simulink subsystem "REGISTERS_10_SS"  (R2022a)
settings: Solver=VariableStepAuto  StartTime=0.0  StopTime=10.0  RelTol=1e-3
libraries: hdlBasic x6395
(part 1 of 23)
settings Model: Creator=sebas  LastModifiedBy=viktor

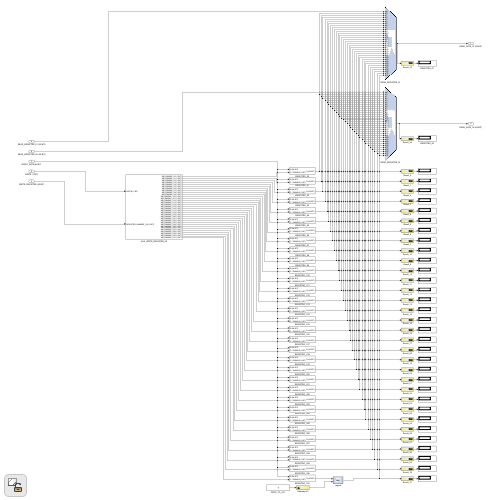
[thumbnail: Simulink's stored preview of the top-level diagram]
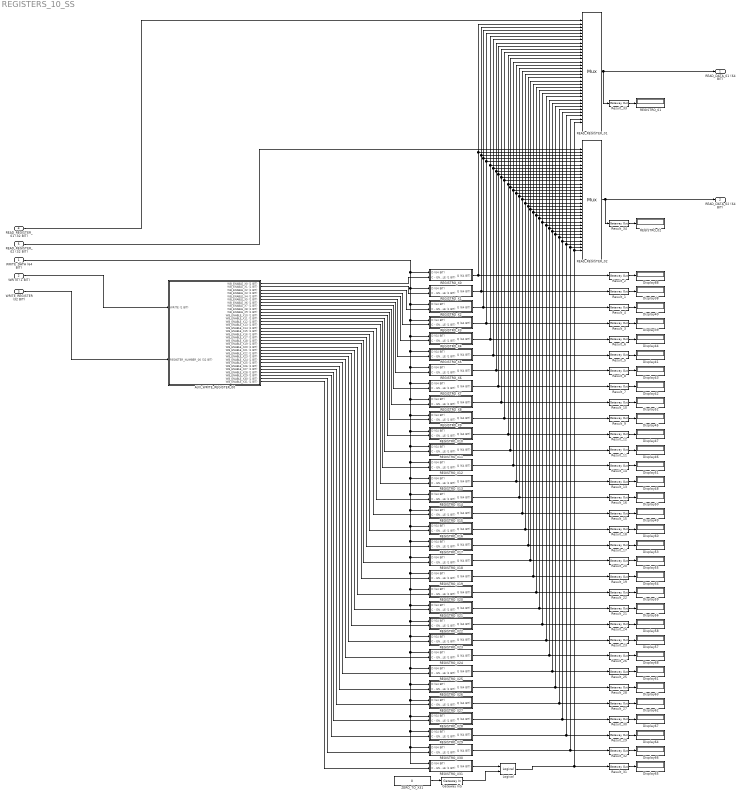
== system REGISTERS_10_SS ==
  WRITE_DATA (64 BIT) : Inport
  WRITE (1 BIT) : Inport  Port=2
  WRITE_REGISTER (32 BIT) : Inport  Port=3
  READ_REGISTER_01 (32 BIT) : Inport  Port=4
  READ_REGISTER_02 (32 BIT) : Inport  Port=5
  AUX_WRITE_REGISTER_00 : Subsystem
  Display{38..68,88} (32 alike) : Display
      settings: Format=decimal (Stored Integer)
  Gateway In5 : hdlBasic/Gateway In  gui_display_data_type=Fixed-point  arith_type=Signed (2's comp)  n_bits=64  bin_pt=0  preci_type=Single  exp_width=8  frac_width=24  rows=1  columns=1  quantization="Round  (unbiased: +/- Inf)"  overflow=Saturate  period=1  UseAsADC=off  ADCChannel='1'  interface=None  automatic_assignment=on  address_offset=hex2dec('00')  intf_name=''  intf_description=''  default_value=0  timing_constraint=None  locs_specified=off  LOCs={}  io_standard={}  inherit_from_input=off  hdl_port=on  XmcBlockStatus=1  maskContainerNames=group4  block_type=gatewayin  block_config=sysgen:gateway_in_config  block_width_w=590  block_height_w=620  block_width=640  block_height=850
  Logical : hdlBasic/Logical  logical_function=AND  inputs=2  en=off  latency=0  precision=Full  arith_type=Unsigned  n_bits=16  bin_pt=0  align_bp=on  overflow=[]  quantization=[]  XmcBlockStatus=1  maskContainerNames=tabcontainer1  block_type=logical  block_config=sysgen:Logical_config
  READ_REGISTER_01 : hdlBasic/Mux  inputs=32  en=off  latency=0  precision=Full  arith_type=Unsigned  n_bits=16  bin_pt=14  quantization=Truncate  overflow=Wrap  XmcBlockStatus=1  maskContainerNames=tabcontainer1  block_type=mux  block_config=sysgen:Mux_config
  READ_REGISTER_02 : hdlBasic/Mux  inputs=32  en=off  latency=0  precision=Full  arith_type=Unsigned  n_bits=16  bin_pt=14  quantization=Truncate  overflow=Wrap  XmcBlockStatus=1  maskContainerNames=tabcontainer1  block_type=mux  block_config=sysgen:Mux_config
  REGISTRO_01 : Display
      settings: Format=decimal (Stored Integer)
  REGISTRO_02 : Display
      settings: Format=decimal (Stored Integer)
  REGISTRO_X0 : Subsystem
  REGISTRO_X1 : Subsystem
  REGISTRO_X10 : Subsystem
  REGISTRO_X11 : Subsystem
  REGISTRO_X12 : Subsystem
  REGISTRO_X13 : Subsystem
  REGISTRO_X14 : Subsystem
  REGISTRO_X15 : Subsystem
  REGISTRO_X16 : Subsystem
  REGISTRO_X17 : Subsystem
  REGISTRO_X18 : Subsystem
  REGISTRO_X19 : Subsystem
  REGISTRO_X2 : Subsystem
  REGISTRO_X20 : Subsystem
  REGISTRO_X21 : Subsystem
  REGISTRO_X22 : Subsystem
  REGISTRO_X23 : Subsystem
  REGISTRO_X24 : Subsystem
  REGISTRO_X25 : Subsystem
  REGISTRO_X26 : Subsystem
  REGISTRO_X27 : Subsystem
  REGISTRO_X28 : Subsystem
  REGISTRO_X29 : Subsystem
  REGISTRO_X3 : Subsystem
  REGISTRO_X30 : Subsystem
  REGISTRO_X31 : Subsystem
  REGISTRO_X4 : Subsystem
  REGISTRO_X5 : Subsystem
  REGISTRO_X6 : Subsystem
  REGISTRO_X7 : Subsystem
  REGISTRO_X8 : Subsystem
  REGISTRO_X9 : Subsystem
  Result_{1..34} (34 alike) : hdlBasic/Gateway Out  inherit_from_input=off  hdl_port=on  rows=1  columns=1  UseAsDAC=off  DACChannel='1'  interface=None  automatic_assignment=on  address_offset=hex2dec('00')  intf_name=''  intf_description=''  timing_constraint=None  locs_specified=off  LOCs={}  io_standard={}  XmcBlockStatus=1  maskContainerNames=group4  block_type=gatewayout  block_config=sysgen:gateway_out_config  block_width_w=590  block_height_w=620  block_width=620  block_height=750
  ZERO_TO_X31 : Constant  Value=0
  READ_DATA_01 (64 BIT) : Outport
  READ_DATA_02 (64 BIT) : Outport  Port=2
  wires:
  REGISTRO_X11/1(Q (64 BIT)) -> Result_11/1, READ_REGISTER_02/13, READ_REGISTER_01/13
  AUX_WRITE_REGISTER_00/26(WB_ENABLE_X25 (1 BIT)) -> REGISTRO_X25/2(C - ENABLE (1 BIT))
  REGISTRO_X14/1(Q (64 BIT)) -> Result_16/1, READ_REGISTER_02/16, READ_REGISTER_01/16
  REGISTRO_X2/1(Q (64 BIT)) -> Result_4/1, READ_REGISTER_02/4, READ_REGISTER_01/4
  REGISTRO_X13/1(Q (64 BIT)) -> Result_13/1, READ_REGISTER_02/15, READ_REGISTER_01/15
  AUX_WRITE_REGISTER_00/10(WB_ENABLE_X9 (1 BIT)) -> REGISTRO_X9/2(C - ENABLE (1 BIT))
  REGISTRO_X1/1(Q (64 BIT)) -> Result_1/1, READ_REGISTER_02/3, READ_REGISTER_01/3
  AUX_WRITE_REGISTER_00/17(WB_ENABLE_X16 (1 BIT)) -> REGISTRO_X16/2(C - ENABLE (1 BIT))
  Result_7/1 -> Display42/1
  ZERO_TO_X31/1 -> Gateway In5/1
  Gateway In5/1 -> Logical/2
  REGISTRO_X8/1(Q (64 BIT)) -> Result_10/1, READ_REGISTER_02/10, READ_REGISTER_01/10
  AUX_WRITE_REGISTER_00/13(WB_ENABLE_X12 (1 BIT)) -> REGISTRO_X12/2(C - ENABLE (1 BIT))
  Result_28/1 -> Display63/1
  WRITE_DATA (64 BIT)/1 -> REGISTRO_X0/1(D (64 BIT)), REGISTRO_X1/1(D (64 BIT)), REGISTRO_X2/1(D (64 BIT)), REGISTRO_X3/1(D (64 BIT)), REGISTRO_X4/1(D (64 BIT)), REGISTRO_X30/1(D (64 BIT)), REGISTRO_X31/1(D (64 BIT)), REGISTRO_X29/1(D (64 BIT)), REGISTRO_X28/1(D (64 BIT)), REGISTRO_X27/1(D (64 BIT)), REGISTRO_X26/1(D (64 BIT)), REGISTRO_X25/1(D (64 BIT)), REGISTRO_X24/1(D (64 BIT)), REGISTRO_X23/1(D (64 BIT)), REGISTRO_X22/1(D (64 BIT)), REGISTRO_X21/1(D (64 BIT)), REGISTRO_X20/1(D (64 BIT)), REGISTRO_X19/1(D (64 BIT)), REGISTRO_X18/1(D (64 BIT)), REGISTRO_X17/1(D (64 BIT)), REGISTRO_X16/1(D (64 BIT)), REGISTRO_X15/1(D (64 BIT)), REGISTRO_X14/1(D (64 BIT)), REGISTRO_X13/1(D (64 BIT)), REGISTRO_X12/1(D (64 BIT)), REGISTRO_X11/1(D (64 BIT)), REGISTRO_X10/1(D (64 BIT)), REGISTRO_X9/1(D (64 BIT)), REGISTRO_X8/1(D (64 BIT)), REGISTRO_X7/1(D (64 BIT)), REGISTRO_X6/1(D (64 BIT)), REGISTRO_X5/1(D (64 BIT))
  Result_24/1 -> Display58/1
  AUX_WRITE_REGISTER_00/32(WB_ENABLE_X31 (1 BIT)) -> REGISTRO_X31/2(C - ENABLE (1 BIT))
  REGISTRO_X23/1(Q (64 BIT)) -> Result_23/1, READ_REGISTER_02/25, READ_REGISTER_01/25
  REGISTRO_X0/1(Q (64 BIT)) -> Result_2/1, READ_REGISTER_02/2, READ_REGISTER_01/2
  AUX_WRITE_REGISTER_00/21(WB_ENABLE_X20 (1 BIT)) -> REGISTRO_X20/2(C - ENABLE (1 BIT))
  Result_25/1 -> Display61/1
  REGISTRO_X12/1(Q (64 BIT)) -> Result_14/1, READ_REGISTER_02/14, READ_REGISTER_01/14
  AUX_WRITE_REGISTER_00/20(WB_ENABLE_X19 (1 BIT)) -> REGISTRO_X19/2(C - ENABLE (1 BIT))
  REGISTRO_X21/1(Q (64 BIT)) -> Result_21/1, READ_REGISTER_02/23, READ_REGISTER_01/23
  REGISTRO_X28/1(Q (64 BIT)) -> Result_30/1, READ_REGISTER_02/30, READ_REGISTER_01/30
  Result_5/1 -> Display41/1
  Logical/1 -> Result_31/1, READ_REGISTER_02/33, READ_REGISTER_01/33
  REGISTRO_X5/1(Q (64 BIT)) -> Result_5/1, READ_REGISTER_02/7, READ_REGISTER_01/7
  WRITE (1 BIT)/1 -> AUX_WRITE_REGISTER_00/1(WRITE (1 BIT))
  AUX_WRITE_REGISTER_00/24(WB_ENABLE_X23 (1 BIT)) -> REGISTRO_X23/2(C - ENABLE (1 BIT))
  AUX_WRITE_REGISTER_00/19(WB_ENABLE_X18 (1 BIT)) -> REGISTRO_X18/2(C - ENABLE (1 BIT))
  Result_12/1 -> Display47/1
  REGISTRO_X15/1(Q (64 BIT)) -> Result_15/1, READ_REGISTER_02/17, READ_REGISTER_01/17
  REGISTRO_X29/1(Q (64 BIT)) -> Result_29/1, READ_REGISTER_02/31, READ_REGISTER_01/31
  AUX_WRITE_REGISTER_00/29(WB_ENABLE_X28 (1 BIT)) -> REGISTRO_X28/2(C - ENABLE (1 BIT))
  REGISTRO_X31/1(Q (64 BIT)) -> Logical/1
  AUX_WRITE_REGISTER_00/16(WB_ENABLE_X15 (1 BIT)) -> REGISTRO_X15/2(C - ENABLE (1 BIT))
  AUX_WRITE_REGISTER_00/18(WB_ENABLE_X17 (1 BIT)) -> REGISTRO_X17/2(C - ENABLE (1 BIT))
  AUX_WRITE_REGISTER_00/28(WB_ENABLE_X27 (1 BIT)) -> REGISTRO_X27/2(C - ENABLE (1 BIT))
  REGISTRO_X3/1(Q (64 BIT)) -> Result_3/1, READ_REGISTER_02/5, READ_REGISTER_01/5
  AUX_WRITE_REGISTER_00/31(WB_ENABLE_X30 (1 BIT)) -> REGISTRO_X30/2(C - ENABLE (1 BIT))
  AUX_WRITE_REGISTER_00/12(WB_ENABLE_X11 (1 BIT)) -> REGISTRO_X11/2(C - ENABLE (1 BIT))
  REGISTRO_X19/1(Q (64 BIT)) -> Result_19/1, READ_REGISTER_02/21, READ_REGISTER_01/21
  AUX_WRITE_REGISTER_00/27(WB_ENABLE_X26 (1 BIT)) -> REGISTRO_X26/2(C - ENABLE (1 BIT))
  Result_31/1 -> Display65/1
  REGISTRO_X30/1(Q (64 BIT)) -> Result_32/1, READ_REGISTER_02/32, READ_REGISTER_01/32
  Result_23/1 -> Display57/1
  AUX_WRITE_REGISTER_00/11(WB_ENABLE_X10 (1 BIT)) -> REGISTRO_X10/2(C - ENABLE (1 BIT))
  Result_18/1 -> Display60/1
  Result_6/1 -> Display44/1
  Result_22/1 -> Display59/1
  REGISTRO_X20/1(Q (64 BIT)) -> Result_22/1, READ_REGISTER_02/22, READ_REGISTER_01/22
  Result_26/1 -> Display68/1
  REGISTRO_X18/1(Q (64 BIT)) -> Result_20/1, READ_REGISTER_02/20, READ_REGISTER_01/20
  Result_33/1 -> REGISTRO_01/1
  REGISTRO_X6/1(Q (64 BIT)) -> Result_8/1, READ_REGISTER_02/8, READ_REGISTER_01/8
  Result_19/1 -> Display54/1
  REGISTRO_X17/1(Q (64 BIT)) -> Result_17/1, READ_REGISTER_02/19, READ_REGISTER_01/19
  Result_21/1 -> Display56/1
  AUX_WRITE_REGISTER_00/15(WB_ENABLE_X14 (1 BIT)) -> REGISTRO_X14/2(C - ENABLE (1 BIT))
  Result_29/1 -> Display64/1
  REGISTRO_X26/1(Q (64 BIT)) -> Result_28/1, READ_REGISTER_02/28, READ_REGISTER_01/28
  REGISTRO_X27/1(Q (64 BIT)) -> Result_27/1, READ_REGISTER_02/29, READ_REGISTER_01/29
  REGISTRO_X25/1(Q (64 BIT)) -> Result_25/1, READ_REGISTER_02/27, READ_REGISTER_01/27
  Result_15/1 -> Display49/1
  REGISTRO_X24/1(Q (64 BIT)) -> Result_26/1, READ_REGISTER_02/26, READ_REGISTER_01/26
  READ_REGISTER_02/1 -> Result_34/1, READ_DATA_02 (64 BIT)/1
  Result_14/1 -> Display51/1
  Result_27/1 -> Display62/1
  REGISTRO_X7/1(Q (64 BIT)) -> Result_7/1, READ_REGISTER_02/9, READ_REGISTER_01/9
  Result_4/1 -> Display40/1
  REGISTRO_X4/1(Q (64 BIT)) -> Result_6/1, READ_REGISTER_02/6, READ_REGISTER_01/6
  Result_17/1 -> Display53/1
  Result_16/1 -> Display50/1
  Result_20/1 -> Display55/1
  Result_32/1 -> Display66/1
  REGISTRO_X9/1(Q (64 BIT)) -> Result_9/1, READ_REGISTER_02/11, READ_REGISTER_01/11
  Result_30/1 -> Display67/1
  READ_REGISTER_02 (32 BIT)/1 -> READ_REGISTER_02/1
  Result_3/1 -> Display39/1
  AUX_WRITE_REGISTER_00/3(WB_ENABLE_X2 (1 BIT)) -> REGISTRO_X2/2(C - ENABLE (1 BIT))
  Result_10/1 -> Display52/1
  REGISTRO_X10/1(Q (64 BIT)) -> Result_12/1, READ_REGISTER_02/12, READ_REGISTER_01/12
  AUX_WRITE_REGISTER_00/4(WB_ENABLE_X3 (1 BIT)) -> REGISTRO_X3/2(C - ENABLE (1 BIT))
  Result_1/1 -> Display38/1
  REGISTRO_X16/1(Q (64 BIT)) -> Result_18/1, READ_REGISTER_02/18, READ_REGISTER_01/18
  Result_2/1 -> Display88/1
  AUX_WRITE_REGISTER_00/2(WB_ENABLE_X1 (1 BIT)) -> REGISTRO_X1/2(C - ENABLE (1 BIT))
  AUX_WRITE_REGISTER_00/14(WB_ENABLE_X13 (1 BIT)) -> REGISTRO_X13/2(C - ENABLE (1 BIT))
  AUX_WRITE_REGISTER_00/6(WB_ENABLE_X5 (1 BIT)) -> REGISTRO_X5/2(C - ENABLE (1 BIT))
  Result_13/1 -> Display48/1
  AUX_WRITE_REGISTER_00/1(WB_ENABLE_X0 (1 BIT)) -> REGISTRO_X0/2(C - ENABLE (1 BIT))
  Result_9/1 -> Display45/1
  READ_REGISTER_01/1 -> Result_33/1, READ_DATA_01 (64 BIT)/1
  REGISTRO_X22/1(Q (64 BIT)) -> Result_24/1, READ_REGISTER_02/24, READ_REGISTER_01/24
  WRITE_REGISTER (32 BIT)/1 -> AUX_WRITE_REGISTER_00/2(REGISTER_NUMBER_00 (32 BIT))
  AUX_WRITE_REGISTER_00/9(WB_ENABLE_X8 (1 BIT)) -> REGISTRO_X8/2(C - ENABLE (1 BIT))
  AUX_WRITE_REGISTER_00/22(WB_ENABLE_X21 (1 BIT)) -> REGISTRO_X21/2(C - ENABLE (1 BIT))
  Result_34/1 -> REGISTRO_02/1
  AUX_WRITE_REGISTER_00/25(WB_ENABLE_X24 (1 BIT)) -> REGISTRO_X24/2(C - ENABLE (1 BIT))
  Result_8/1 -> Display43/1
  Result_11/1 -> Display46/1
  AUX_WRITE_REGISTER_00/7(WB_ENABLE_X6 (1 BIT)) -> REGISTRO_X6/2(C - ENABLE (1 BIT))
  AUX_WRITE_REGISTER_00/5(WB_ENABLE_X4 (1 BIT)) -> REGISTRO_X4/2(C - ENABLE (1 BIT))
  AUX_WRITE_REGISTER_00/8(WB_ENABLE_X7 (1 BIT)) -> REGISTRO_X7/2(C - ENABLE (1 BIT))
  AUX_WRITE_REGISTER_00/23(WB_ENABLE_X22 (1 BIT)) -> REGISTRO_X22/2(C - ENABLE (1 BIT))
  AUX_WRITE_REGISTER_00/30(WB_ENABLE_X29 (1 BIT)) -> REGISTRO_X29/2(C - ENABLE (1 BIT))
  READ_REGISTER_01 (32 BIT)/1 -> READ_REGISTER_01/1

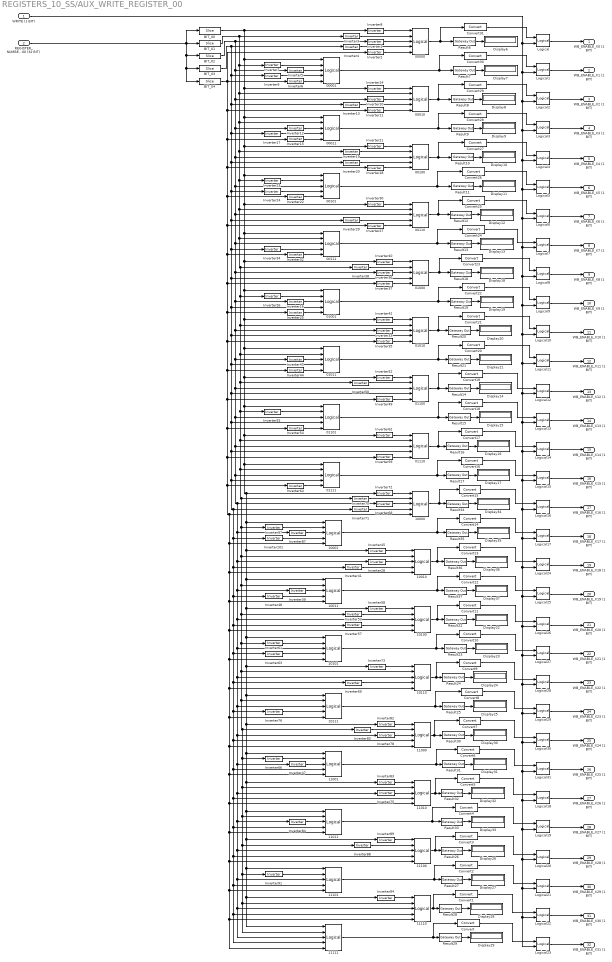
== system REGISTERS_10_SS/AUX_WRITE_REGISTER_00 ==
  WRITE (1 BIT) : Inport
  REGISTER_NUMBER_00 (32 BIT) : Inport  Port=2
  00000 : hdlBasic/Logical  logical_function=AND  inputs=5  en=off  latency=0  precision=Full  arith_type=Unsigned  n_bits=16  bin_pt=0  align_bp=on  overflow=[]  quantization=[]  XmcBlockStatus=1  maskContainerNames=tabcontainer1  block_type=logical  block_config=sysgen:Logical_config
  00001 : hdlBasic/Logical  logical_function=AND  inputs=5  en=off  latency=0  precision=Full  arith_type=Unsigned  n_bits=16  bin_pt=0  align_bp=on  overflow=[]  quantization=[]  XmcBlockStatus=1  maskContainerNames=tabcontainer1  block_type=logical  block_config=sysgen:Logical_config
  00010 : hdlBasic/Logical  logical_function=AND  inputs=5  en=off  latency=0  precision=Full  arith_type=Unsigned  n_bits=16  bin_pt=0  align_bp=on  overflow=[]  quantization=[]  XmcBlockStatus=1  maskContainerNames=tabcontainer1  block_type=logical  block_config=sysgen:Logical_config
  00011 : hdlBasic/Logical  logical_function=AND  inputs=5  en=off  latency=0  precision=Full  arith_type=Unsigned  n_bits=16  bin_pt=0  align_bp=on  overflow=[]  quantization=[]  XmcBlockStatus=1  maskContainerNames=tabcontainer1  block_type=logical  block_config=sysgen:Logical_config
  00100 : hdlBasic/Logical  logical_function=AND  inputs=5  en=off  latency=0  precision=Full  arith_type=Unsigned  n_bits=16  bin_pt=0  align_bp=on  overflow=[]  quantization=[]  XmcBlockStatus=1  maskContainerNames=tabcontainer1  block_type=logical  block_config=sysgen:Logical_config
  00101 : hdlBasic/Logical  logical_function=AND  inputs=5  en=off  latency=0  precision=Full  arith_type=Unsigned  n_bits=16  bin_pt=0  align_bp=on  overflow=[]  quantization=[]  XmcBlockStatus=1  maskContainerNames=tabcontainer1  block_type=logical  block_config=sysgen:Logical_config
  00110 : hdlBasic/Logical  logical_function=AND  inputs=5  en=off  latency=0  precision=Full  arith_type=Unsigned  n_bits=16  bin_pt=0  align_bp=on  overflow=[]  quantization=[]  XmcBlockStatus=1  maskContainerNames=tabcontainer1  block_type=logical  block_config=sysgen:Logical_config
  00111 : hdlBasic/Logical  logical_function=AND  inputs=5  en=off  latency=0  precision=Full  arith_type=Unsigned  n_bits=16  bin_pt=0  align_bp=on  overflow=[]  quantization=[]  XmcBlockStatus=1  maskContainerNames=tabcontainer1  block_type=logical  block_config=sysgen:Logical_config
  01000 : hdlBasic/Logical  logical_function=AND  inputs=5  en=off  latency=0  precision=Full  arith_type=Unsigned  n_bits=16  bin_pt=0  align_bp=on  overflow=[]  quantization=[]  XmcBlockStatus=1  maskContainerNames=tabcontainer1  block_type=logical  block_config=sysgen:Logical_config
  01001 : hdlBasic/Logical  logical_function=AND  inputs=5  en=off  latency=0  precision=Full  arith_type=Unsigned  n_bits=16  bin_pt=0  align_bp=on  overflow=[]  quantization=[]  XmcBlockStatus=1  maskContainerNames=tabcontainer1  block_type=logical  block_config=sysgen:Logical_config
  01010 : hdlBasic/Logical  logical_function=AND  inputs=5  en=off  latency=0  precision=Full  arith_type=Unsigned  n_bits=16  bin_pt=0  align_bp=on  overflow=[]  quantization=[]  XmcBlockStatus=1  maskContainerNames=tabcontainer1  block_type=logical  block_config=sysgen:Logical_config
  01011 : hdlBasic/Logical  logical_function=AND  inputs=5  en=off  latency=0  precision=Full  arith_type=Unsigned  n_bits=16  bin_pt=0  align_bp=on  overflow=[]  quantization=[]  XmcBlockStatus=1  maskContainerNames=tabcontainer1  block_type=logical  block_config=sysgen:Logical_config
  01100 : hdlBasic/Logical  logical_function=AND  inputs=5  en=off  latency=0  precision=Full  arith_type=Unsigned  n_bits=16  bin_pt=0  align_bp=on  overflow=[]  quantization=[]  XmcBlockStatus=1  maskContainerNames=tabcontainer1  block_type=logical  block_config=sysgen:Logical_config
  01101 : hdlBasic/Logical  logical_function=AND  inputs=5  en=off  latency=0  precision=Full  arith_type=Unsigned  n_bits=16  bin_pt=0  align_bp=on  overflow=[]  quantization=[]  XmcBlockStatus=1  maskContainerNames=tabcontainer1  block_type=logical  block_config=sysgen:Logical_config
  01110 : hdlBasic/Logical  logical_function=AND  inputs=5  en=off  latency=0  precision=Full  arith_type=Unsigned  n_bits=16  bin_pt=0  align_bp=on  overflow=[]  quantization=[]  XmcBlockStatus=1  maskContainerNames=tabcontainer1  block_type=logical  block_config=sysgen:Logical_config
  01111 : hdlBasic/Logical  logical_function=AND  inputs=5  en=off  latency=0  precision=Full  arith_type=Unsigned  n_bits=16  bin_pt=0  align_bp=on  overflow=[]  quantization=[]  XmcBlockStatus=1  maskContainerNames=tabcontainer1  block_type=logical  block_config=sysgen:Logical_config
  {10000..10001,10010..10011,10100..10101,10110..10111,11000..11001,11010..11011,11100..11101,11110..11111} (16 alike) : hdlBasic/Logical  logical_function=AND  inputs=5  en=off  latency=0  precision=Full  arith_type=Unsigned  n_bits=16  bin_pt=0  align_bp=on  overflow=[]  quantization=[]  XmcBlockStatus=1  maskContainerNames=tabcontainer1  block_type=logical  block_config=sysgen:Logical_config
  BIT_00 : hdlBasic/Slice  nbits=1  boolean_output=off  mode=Lower Bit Location + Width  bit1=-3  base1=MSB of Input  bit0=0  base0=LSB of Input  XmcBlockStatus=1  maskContainerNames=group1  block_type=slice  block_config=sysgen:Slice_config
  BIT_01 : hdlBasic/Slice  nbits=1  boolean_output=off  mode=Lower Bit Location + Width  bit1=-2  base1=MSB of Input  bit0=1  base0=LSB of Input  XmcBlockStatus=1  maskContainerNames=group1  block_type=slice  block_config=sysgen:Slice_config
  BIT_02 : hdlBasic/Slice  nbits=1  boolean_output=off  mode=Lower Bit Location + Width  bit1=-3  base1=MSB of Input  bit0=2  base0=LSB of Input  XmcBlockStatus=1  maskContainerNames=group1  block_type=slice  block_config=sysgen:Slice_config
  BIT_03 : hdlBasic/Slice  nbits=1  boolean_output=off  mode=Lower Bit Location + Width  bit1=-2  base1=MSB of Input  bit0=3  base0=LSB of Input  XmcBlockStatus=1  maskContainerNames=group1  block_type=slice  block_config=sysgen:Slice_config
  BIT_04 : hdlBasic/Slice  nbits=1  boolean_output=off  mode=Lower Bit Location + Width  bit1=-2  base1=MSB of Input  bit0=4  base0=LSB of Input  XmcBlockStatus=1  maskContainerNames=group1  block_type=slice  block_config=sysgen:Slice_config
  Convert{,1..31} (32 alike) : hdlBasic/Convert  gui_display_data_type=Boolean  arith_type=Boolean  n_bits=16  bin_pt=14  float_type=Single  exp_bits=8  fraction_bits=24  quantization=Truncate  overflow=Wrap  en=off  latency=0  pipeline=off  XmcBlockStatus=1  maskContainerNames=group2  block_type=convert  block_config=sysgen:Convert_config  block_width=595  block_height=885
  Display{6..37} (32 alike) : Display
  Inverter{1..30,32..45,47..50,52..55,57..59,61..64,66,68..73,75..76,78,80,82..84,87..89,91,94,97,101} (80 alike) : hdlBasic/Inverter  en=off  latency=0  XmcBlockStatus=1  maskContainerNames=group2  block_type=inv  block_config=sysgen:Inverter_config
  Logical{,1..31} (32 alike) : hdlBasic/Logical  logical_function=AND  inputs=2  en=off  latency=0  precision=Full  arith_type=Unsigned  n_bits=16  bin_pt=0  align_bp=on  overflow=[]  quantization=[]  XmcBlockStatus=1  maskContainerNames=tabcontainer1  block_type=logical  block_config=sysgen:Logical_config
  Result{6..37} (32 alike) : hdlBasic/Gateway Out  inherit_from_input=off  hdl_port=on  rows=1  columns=1  UseAsDAC=off  DACChannel='1'  interface=None  automatic_assignment=on  address_offset=hex2dec('00')  intf_name=''  intf_description=''  timing_constraint=None  locs_specified=off  LOCs={}  io_standard={}  XmcBlockStatus=1  maskContainerNames=group4  block_type=gatewayout  block_config=sysgen:gateway_out_config  block_width_w=590  block_height_w=620  block_width=620  block_height=750
  WB_ENABLE_X0 (1 BIT) : Outport
  WB_ENABLE_X1 (1 BIT) : Outport  Port=2
  WB_ENABLE_X2 (1 BIT) : Outport  Port=3
  WB_ENABLE_X3 (1 BIT) : Outport  Port=4
  WB_ENABLE_X4 (1 BIT) : Outport  Port=5
  WB_ENABLE_X5 (1 BIT) : Outport  Port=6
  WB_ENABLE_X6 (1 BIT) : Outport  Port=7
  WB_ENABLE_X7 (1 BIT) : Outport  Port=8
  WB_ENABLE_X8 (1 BIT) : Outport  Port=9
  WB_ENABLE_X9 (1 BIT) : Outport  Port=10
  WB_ENABLE_X10 (1 BIT) : Outport  Port=11
  WB_ENABLE_X11 (1 BIT) : Outport  Port=12
  WB_ENABLE_X12 (1 BIT) : Outport  Port=13
  WB_ENABLE_X13 (1 BIT) : Outport  Port=14
  WB_ENABLE_X14 (1 BIT) : Outport  Port=15
  WB_ENABLE_X15 (1 BIT) : Outport  Port=16
  WB_ENABLE_X16 (1 BIT) : Outport  Port=17
  WB_ENABLE_X17 (1 BIT) : Outport  Port=18
  WB_ENABLE_X18 (1 BIT) : Outport  Port=19
  WB_ENABLE_X19 (1 BIT) : Outport  Port=20
  WB_ENABLE_X20 (1 BIT) : Outport  Port=21
  WB_ENABLE_X21 (1 BIT) : Outport  Port=22
  WB_ENABLE_X22 (1 BIT) : Outport  Port=23
  WB_ENABLE_X23 (1 BIT) : Outport  Port=24
  WB_ENABLE_X24 (1 BIT) : Outport  Port=25
  WB_ENABLE_X25 (1 BIT) : Outport  Port=26
  WB_ENABLE_X26 (1 BIT) : Outport  Port=27
  WB_ENABLE_X27 (1 BIT) : Outport  Port=28
  WB_ENABLE_X28 (1 BIT) : Outport  Port=29
  WB_ENABLE_X29 (1 BIT) : Outport  Port=30
  WB_ENABLE_X30 (1 BIT) : Outport  Port=31
  WB_ENABLE_X31 (1 BIT) : Outport  Port=32
  wires:
  Logical3/1 -> WB_ENABLE_X3 (1 BIT)/1
  Inverter44/1 -> 01011/5
  Inverter88/1 -> 11100/2
  Result19/1 -> Display19/1
  Inverter6/1 -> 00001/5
  Convert18/1 -> Logical13/1
  00000/1 -> Result6/1, Convert31/1
  Result28/1 -> Display28/1
  Result7/1 -> Display7/1
  Inverter97/1 -> 10001/2
  Inverter41/1 -> 10010/4
  Convert19/1 -> Logical12/1
  Inverter43/1 -> 01011/3
  Inverter10/1 -> 00010/3
  Logical9/1 -> WB_ENABLE_X9 (1 BIT)/1
  Logical13/1 -> WB_ENABLE_X13 (1 BIT)/1
  Logical14/1 -> WB_ENABLE_X14 (1 BIT)/1
  Logical11/1 -> WB_ENABLE_X11 (1 BIT)/1
  Result22/1 -> Display22/1
  Inverter63/1 -> 10101/4
  Convert8/1 -> Logical29/1
  Inverter16/1 -> 01001/3
  Inverter66/1 -> 11001/2
  Convert5/1 -> Logical18/1
  Result12/1 -> Display12/1
  Inverter80/1 -> 11000/2
  Inverter17/1 -> 00011/4
  Result18/1 -> Display18/1
  Inverter8/1 -> 00000/1
  Result27/1 -> Display27/1
  Inverter34/1 -> 00111/4
  Result36/1 -> Display36/1
  11000/1 -> Result30/1, Convert7/1
  Logical/1 -> WB_ENABLE_X0 (1 BIT)/1
  Logical30/1 -> WB_ENABLE_X24 (1 BIT)/1
  Logical18/1 -> WB_ENABLE_X26 (1 BIT)/1
  Logical20/1 -> WB_ENABLE_X28 (1 BIT)/1
  Logical31/1 -> WB_ENABLE_X25 (1 BIT)/1
  Logical22/1 -> WB_ENABLE_X30 (1 BIT)/1
  Logical29/1 -> WB_ENABLE_X23 (1 BIT)/1
  Inverter38/1 -> 01000/2
  Logical24/1 -> WB_ENABLE_X18 (1 BIT)/1
  Logical1/1 -> WB_ENABLE_X1 (1 BIT)/1
  Inverter47/1 -> 11001/3
  01100/1 -> Result14/1, Convert19/1
  Result35/1 -> Display35/1
  Convert6/1 -> Logical31/1
  Convert4/1 -> Logical19/1
  Inverter83/1 -> 11010/1
  Convert3/1 -> Logical20/1
  10000/1 -> Result34/1, Convert15/1
  Inverter13/1 -> 00010/4
  Inverter75/1 -> 11010/3
  Convert11/1 -> Logical26/1
  Result29/1 -> Display29/1
  Inverter101/1 -> 10001/4
  Inverter72/1 -> 10000/1
  Inverter1/1 -> 00000/3
  Inverter3/1 -> 00000/2
  Convert15/1 -> Logical16/1
  Inverter14/1 -> 00010/1
  Inverter21/1 -> 00100/1
  Convert26/1 -> Logical5/1
  Inverter11/1 -> 00010/5
  Inverter58/1 -> 10100/1
  Result33/1 -> Display33/1
  Inverter36/1 -> 01000/3
  Inverter45/1 -> 10010/1
  Inverter9/1 -> 00001/4
  Inverter68/1 -> 10000/3
  01001/1 -> Result19/1, Convert22/1
  Logical21/1 -> WB_ENABLE_X29 (1 BIT)/1
  Convert9/1 -> Logical28/1
  Inverter25/1 -> 01001/5
  Result10/1 -> Display10/1
  Logical12/1 -> WB_ENABLE_X12 (1 BIT)/1
  Result11/1 -> Display11/1
  Result8/1 -> Display8/1
  Inverter5/1 -> 00001/3
  Inverter15/1 -> 00011/5
  Result25/1 -> Display25/1
  Result37/1 -> Display37/1
  Result16/1 -> Display16/1
  Result14/1 -> Display14/1
  Inverter59/1 -> 01110/5
  Convert14/1 -> Logical17/1
  Convert12/1 -> Logical25/1
  Logical17/1 -> WB_ENABLE_X17 (1 BIT)/1
  Convert10/1 -> Logical27/1
  Convert17/1 -> Logical14/1
  Inverter23/1 -> 00101/2
  Convert23/1 -> Logical8/1
  Convert30/1 -> Logical1/1
  Inverter24/1 -> 00101/4
  10111/1 -> Result25/1, Convert8/1
  Inverter20/1 -> 00100/4
  Inverter53/1 -> 10100/2
  Inverter73/1 -> 10110/1
  Convert22/1 -> Logical9/1
  Inverter7/1 -> 00001/2
  Inverter19/1 -> 00100/2
  01011/1 -> Result21/1, Convert20/1
  Convert13/1 -> Logical24/1
  Inverter84/1 -> 11011/3
  Result20/1 -> Display20/1
  Inverter48/1 -> 10011/4
  Inverter55/1 -> 01101/2
  Logical15/1 -> WB_ENABLE_X15 (1 BIT)/1
  10110/1 -> Result24/1, Convert9/1
  Result23/1 -> Display23/1
  Convert20/1 -> Logical11/1
  01000/1 -> Result18/1, Convert23/1
  11111/1 -> Result29/1, Convert/1
  Result17/1 -> Display17/1
  11110/1 -> Result28/1, Convert1/1
  01110/1 -> Result16/1, Convert17/1
  Inverter2/1 -> 00000/5
  Convert21/1 -> Logical10/1
  Inverter12/1 -> 00011/3
  Inverter27/1 -> 00110/5
  Convert1/1 -> Logical22/1
  Inverter37/1 -> 01000/5
  11101/1 -> Result27/1, Convert2/1
  Inverter32/1 -> 00111/5
  Inverter76/1 -> 10111/4
  Inverter62/1 -> 01110/1
  Inverter22/1 -> 00101/5
  01101/1 -> Result15/1, Convert18/1
  00100/1 -> Result10/1, Convert27/1
  10010/1 -> Result36/1, Convert13/1
  Result34/1 -> Display34/1
  Result9/1 -> Display9/1
  Inverter40/1 -> 01000/1
  Logical2/1 -> WB_ENABLE_X2 (1 BIT)/1
  Inverter87/1 -> 10001/3
  Inverter18/1 -> 00100/5
  Result15/1 -> Display15/1
  Inverter4/1 -> 00000/4
  01010/1 -> Result20/1, Convert21/1
  Inverter64/1 -> 01111/5
  Logical23/1 -> WB_ENABLE_X31 (1 BIT)/1
  Result24/1 -> Display24/1
  Inverter49/1 -> 01100/5
  00001/1 -> Result7/1, Convert30/1
  10101/1 -> Result23/1, Convert10/1
  Result32/1 -> Display32/1
  Inverter50/1 -> 01100/2
  REGISTER_NUMBER_00 (32 BIT)/1 -> BIT_01/1, BIT_04/1, BIT_03/1, BIT_02/1, BIT_00/1
  Inverter42/1 -> 01010/1
  Convert/1 -> Logical23/1
  Inverter71/1 -> 10000/4
  Inverter91/1 -> 11101/2
  Inverter70/1 -> 10000/2
  Convert31/1 -> Logical/1
  10100/1 -> Result22/1, Convert11/1
  Inverter28/1 -> 10010/3
  Inverter78/1 -> 11000/3
  Logical4/1 -> WB_ENABLE_X4 (1 BIT)/1
  Inverter89/1 -> 11100/1
  Inverter39/1 -> 10011/3
  Inverter82/1 -> 11000/1
  11011/1 -> Result33/1, Convert4/1
  Logical7/1 -> WB_ENABLE_X7 (1 BIT)/1
  Logical28/1 -> WB_ENABLE_X22 (1 BIT)/1
  Convert24/1 -> Logical7/1
  Inverter94/1 -> 11110/1
  10011/1 -> Result37/1, Convert12/1
  Convert16/1 -> Logical15/1
  Logical10/1 -> WB_ENABLE_X10 (1 BIT)/1
  Result21/1 -> Display21/1
  Logical19/1 -> WB_ENABLE_X27 (1 BIT)/1
  Inverter69/1 -> 10110/4
  Inverter61/1 -> 10101/2
  00010/1 -> Result8/1, Convert29/1
  00111/1 -> Result13/1, Convert24/1
  Result30/1 -> Display30/1
  Inverter29/1 -> 00110/4
  11100/1 -> Result26/1, Convert3/1
  Logical27/1 -> WB_ENABLE_X21 (1 BIT)/1
  BIT_02/1 -> Inverter1/1, Inverter5/1, 00100/3, 00101/3, 00110/3, 00111/3, Inverter36/1, Inverter16/1, Inverter33/1, Inverter43/1, 01100/3, 01101/3, Inverter68/1, Inverter87/1, 10100/3, 10101/3, 10110/3, 10111/3, Inverter78/1, Inverter47/1, Inverter75/1, Inverter84/1, 11100/3, 11101/3, 11111/3, 11110/3, Inverter39/1, Inverter28/1, 01111/3, 01110/3, Inverter12/1, Inverter10/1
  11001/1 -> Result31/1, Convert6/1
  Convert25/1 -> Logical6/1
  Logical5/1 -> WB_ENABLE_X5 (1 BIT)/1
  Inverter30/1 -> 00110/1
  Result6/1 -> Display6/1
  01111/1 -> Result17/1, Convert16/1
  10001/1 -> Result35/1, Convert14/1
  Inverter35/1 -> 01010/5
  00110/1 -> Result12/1, Convert25/1
  Inverter57/1 -> 10100/4
  Inverter54/1 -> 01101/5
  11010/1 -> Result32/1, Convert5/1
  Convert29/1 -> Logical2/1
  Inverter33/1 -> 01010/3
  BIT_04/1 -> Inverter6/1, Inverter2/1, Inverter11/1, Inverter22/1, Inverter27/1, Inverter32/1, Inverter37/1, 10000/5, 10001/5, 10010/5, 10011/5, 10101/5, 10111/5, 11111/5, 11110/5, 11101/5, 11100/5, 11011/5, 11010/5, 11001/5, 11000/5, 10110/5, 10100/5, Inverter64/1, Inverter59/1, Inverter54/1, Inverter49/1, Inverter44/1, Inverter35/1, Inverter25/1, Inverter18/1, Inverter15/1
  Logical8/1 -> WB_ENABLE_X8 (1 BIT)/1
  Result26/1 -> Display26/1
  Inverter52/1 -> 01100/1
  Inverter26/1 -> 01001/2
  Convert28/1 -> Logical3/1
  BIT_01/1 -> Inverter3/1, Inverter7/1, 00110/2, Inverter38/1, 01010/2, 01110/2, Inverter70/1, Inverter97/1, 10110/2, Inverter80/1, 11010/2, 11110/2, 11111/2, Inverter91/1, Inverter88/1, 11011/2, Inverter66/1, 10111/2, Inverter61/1, Inverter53/1, 10011/2, 10010/2, 01111/2, Inverter55/1, Inverter50/1, 01011/2, Inverter26/1, 00111/2, Inverter23/1, Inverter19/1, 00011/2, 00010/2
  Logical6/1 -> WB_ENABLE_X6 (1 BIT)/1
  Logical26/1 -> WB_ENABLE_X20 (1 BIT)/1
  Result13/1 -> Display13/1
  BIT_03/1 -> Inverter4/1, Inverter9/1, Inverter13/1, Inverter17/1, 01000/4, 01001/4, 01010/4, 01011/4, Inverter71/1, Inverter101/1, Inverter41/1, Inverter48/1, 11000/4, 11001/4, 11010/4, 11011/4, 11111/4, 11110/4, 11101/4, 11100/4, Inverter76/1, Inverter69/1, Inverter63/1, Inverter57/1, 01111/4, 01110/4, 01101/4, 01100/4, Inverter34/1, Inverter29/1, Inverter24/1, Inverter20/1
  00011/1 -> Result9/1, Convert28/1
  00101/1 -> Result11/1, Convert26/1
  Logical25/1 -> WB_ENABLE_X19 (1 BIT)/1
  Convert27/1 -> Logical4/1
  BIT_00/1 -> Inverter8/1, 00001/1, Inverter14/1, 00011/1, Inverter21/1, 00101/1, Inverter30/1, 00111/1, Inverter40/1, Inverter42/1, Inverter52/1, Inverter62/1, Inverter72/1, 10001/1, Inverter45/1, 10011/1, Inverter58/1, 10101/1, Inverter73/1, 10111/1, Inverter82/1, Inverter83/1, Inverter89/1, Inverter94/1, 11111/1, 11101/1, 11011/1, 11001/1, 01111/1, 01101/1, 01011/1, 01001/1
  Convert2/1 -> Logical21/1
  Result31/1 -> Display31/1
  WRITE (1 BIT)/1 -> Logical/2, Logical1/2, Logical2/2, Logical3/2, Logical4/2, Logical5/2, Logical6/2, Logical7/2, Logical8/2, Logical9/2, Logical10/2, Logical11/2, Logical12/2, Logical14/2, Logical16/2, Logical17/2, Logical24/2, Logical25/2, Logical26/2, Logical27/2, Logical28/2, Logical29/2, Logical31/2, Logical18/2, Logical19/2, Logical22/2, Logical23/2, Logical21/2, Logical20/2, Logical30/2, Logical15/2, Logical13/2
  Convert7/1 -> Logical30/1
  Logical16/1 -> WB_ENABLE_X16 (1 BIT)/1
